simulink model "Single_Phase_H_Bridge_Inverter_14_04"  (R2020b)
settings: Solver=VariableStepAuto  StartTime=0.0  StopTime=.04  RelTol=1e-3
libraries: powerlib x14
settings Model: Creator=ADHIP  LastModifiedBy=ADHIP

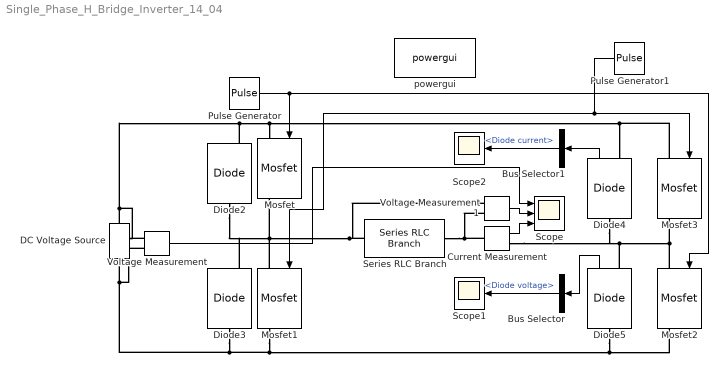
== system Single_Phase_H_Bridge_Inverter_14_04 ==
  Bus Selector : BusSelector  OutputSignals=Diode voltage
  Bus Selector1 : BusSelector  OutputSignals=Diode current
  Current Measurement : powerlib/Measurements/Current Measurement  PhasorSimulation=off  OutputType=Complex  PSBequivalent=0
  DC Voltage Source : powerlib/Electrical Sources/DC Voltage Source  Amplitude=20  Measurements=None
  Diode{2..5} (4 alike) : powerlib/Power Electronics/Diode  Ron=0.001  Lon=0  Vf=0.8  IC=0  UseSnubber=0  Rs=500  Cs=250e-9  Measurements=on
  Mosfet{,1..3} (4 alike) : powerlib/Power Electronics/Mosfet  Ron=0.1  Lon=0  Rd=0.01  Vfd=0  IC=0  Rs=1e5  Cs=inf  Measurements=on
  Pulse Generator : DiscretePulseGenerator  PulseType=Time based  Period=1/50  PulseWidth=50
  Pulse Generator1 : DiscretePulseGenerator  PulseType=Time based  Period=1/50  PulseWidth=50  PhaseDelay=.01
  Scope : Scope  NumInputPorts=3
  Scope1 : Scope
  Scope2 : Scope
  Series RLC Branch : powerlib/Elements/Series RLC Branch  LConnTagsString=__new0  RConnTagsString=__new0  BranchType=RL  Resistance=10  Inductance=1e-3  SetiL0=off  InitialCurrent=0  Capacitance=1e-6  Setx0=off  InitialVoltage=0  Measurements=None
  Voltage Measurement : powerlib/Measurements/Voltage Measurement  PhasorSimulation=off  OutputType=Complex  PSBequivalent=0
  Voltage Measurement1 : powerlib/Measurements/Voltage Measurement  PhasorSimulation=off  OutputType=Complex  PSBequivalent=0
  powergui : powerlib/powergui  Priority=1  SimulationMode=Continuous  SampleTime=50e-6  frequency=60  Iterations=50  frequencyindice=0  Pbase=100e6  ErrMax=1e-4  UnitsV=kV  UnitsW=MW  buscounter=0  FunctionMessages=off  echomessages=off  EnableUseOfTLC=off  CurrentSourceSwitches=off  DisableSnubberDevices=off  DisableRonSwitches=off  DisableVfSwitches=off  DisplayEquations=off  AutomaticDiscreteSolvers=off  SolverType=Tustin/Backward Euler (TBE)  Interpol=off  ExternalGateDelay=off  methode=off  Ts=100  x0status=blocks  SPID=on  SwTol=0  HookPort=off  NonlinearTolerance=1e-4  nMaxIteration=100  ContinueOnMaxIteration=off  RestoreLinks=warning  ResistiveCurrentMeasurement=off  Frange=[0:2:500]  Ylog=off  Xlog=on  ShowGrid=off  save=off  variable=ZData  structure=0  ZoomFFT=off  StartTime=0.0  cycles=1  DisplayStyle=1  fundamental=60  FreqAxis=off  MaxFrequency=1000  frequencyindicesteady=1  RmsSteady=1  display=off
  wires:
  Voltage Measurement/1 -> Scope/1
  Voltage Measurement1/1 -> Scope/2
  Current Measurement/1 -> Scope/3
  Pulse Generator/1 -> Mosfet/1, Mosfet2/1
  Pulse Generator1/1 -> Mosfet3/1, Mosfet1/1
  Bus Selector/1 -> Scope1/1  "<Diode voltage>"
  Bus Selector1/1 -> Scope2/1  "<Diode current>"
  Diode4/1 -> Bus Selector1/1
  Diode5/1 -> Bus Selector/1
  connections:
  DC Voltage Source/RConn1 -- Diode2/RConn1 -- Mosfet3/LConn1 -- Diode4/RConn1 -- Mosfet/LConn1 -- Voltage Measurement/LConn1
  Mosfet1/RConn1 -- Diode5/LConn1 -- Mosfet2/RConn1 -- Voltage Measurement/LConn2 -- DC Voltage Source/LConn1 -- Diode3/LConn1
  Current Measurement/LConn1 -- Series RLC Branch/RConn1 -- Voltage Measurement1/LConn2
  Mosfet1/LConn1 -- Diode2/LConn1 -- Diode3/RConn1 -- Series RLC Branch/LConn1 -- Voltage Measurement1/LConn1 -- Mosfet/RConn1
  Mosfet2/LConn1 -- Diode4/LConn1 -- Current Measurement/RConn1 -- Diode5/RConn1 -- Mosfet3/RConn1
